simulink model "quanser_aero_dynamics4"  (R2021a)
settings: Solver=ode1  StartTime=0.0  StopTime=inf  FixedStep=0.002  RelTol=1e-3  EnableMultiTasking=on
PreLoadFcn:
  | quanser_aero_pd_design;
undefined symbols (not defined in the file): Kc, Kr
libraries: quanser_aero x1
settings Model: SimulationMode=external  ExtModeTrigDuration=15000  Creator=MLevis  LastModifiedBy=Mechatronics
settings SolverCC: AlgebraicLoopSolver=TrustRegion  PositivePriorityOrder=on
settings DataIOCC: LimitDataPoints=on  SaveFormat=Array  ReturnWorkspaceOutputs=off
settings DebuggingCC: SolverPrmCheckMsg=warning  SFUnexpectedBacktrackingDiag=warning  SFNoUnconditionalDefaultTransitionDiag=warning  SFExecutionAtInitializationDiag=none  SFMachineParentedDataDiag=warning  ArithmeticOperatorsInVariantConditions=warning
settings ModelReferenceCC: PropagateSignalLabelsOutOfModel=off
settings SFSimCC: SimUseLocalCustomCode=off  CustomCodeUndefinedFunction=UseInterfaceOnly
settings RTWCC: Description=QUARC Win64 Target Using Toolchain  SystemTargetFile=quarc_win64.tlc  TemplateMakefile=quarc_default_tmf  RTWUseLocalCustomCode=off  Toolchain=QUARC win64 | nmake (64-bit Windows)  BuildConfiguration=Faster Runs
settings CodeAppCC: StateflowObjectComments=on
settings STFCustomTargetCC: ConcurrentExecutionCompliant=on  SystemTargetFile=quarc_win64.tlc
settings GRTTargetCC: TargetLangStandard=C89/C90 (ANSI)  ParMdlRefBuildCompliant=off  CompOptLevelCompliant=off  CombineOutputUpdateFcns=off  MatFileLogging=off  CPPClassGenCompliant=off  GRTInterface=on  ExtMode=on  ExtModeMexFile=quarc_comm
settings ConfigComp: CovMetricSettings=dw  CovSaveCumulativeToWorkspaceVar=on  CovSaveSingleToWorkspaceVar=on  CovExternalEMLEnable=off  CovSFcnEnable=off

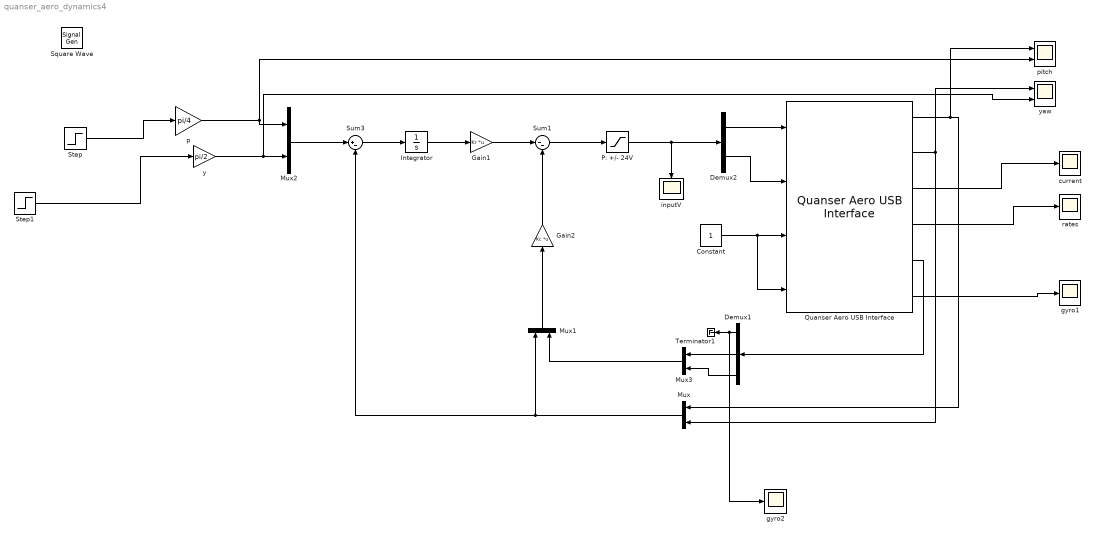
== system quanser_aero_dynamics4 ==
  Constant : Constant
  Demux1 : Demux  Outputs=3
  Demux2 : Demux  Outputs=2
  Gain1 : Gain  Gain=Kr  Multiplication=Matrix(K*u)
  Gain2 : Gain  Gain=Kc  Multiplication=Matrix(K*u)
  Integrator : Integrator
  Mux{,1..3} (4 alike) : Mux  Inputs=2
  P: +/- 24V : Saturate  UpperLimit=24  LowerLimit=-24
  Quanser Aero USB Interface : quanser_aero/Quanser Aero USB Interface  SystemSampleTime=-1  VariantActivationTime=update diagram  Latency=0  AutoFrameSizeCalculation=off
  "Square Wave " : SignalGenerator  WaveForm=square  Frequency=1/8
  Step : Step  Time=0  SampleTime=0
  Step1 : Step  Time=0  SampleTime=0
  Sum1 : Sum  Inputs=|--
  Sum3 : Sum  Inputs=|+-
  Terminator1 : Terminator
  current : Scope
  gyro1 : Scope
  gyro2 : Scope
  inputV : Scope
  p : Gain  Gain=pi/4
  pitch : Scope  NumInputPorts=2
  rates : Scope
  y : Gain  Gain=pi/2
  yaw : Scope  NumInputPorts=2
  wires:
  Mux2/1 -> Sum3/1
  Quanser Aero USB Interface/5 -> Demux1/1
  Quanser Aero USB Interface/4 -> rates/1
  Quanser Aero USB Interface/3 -> current/1
  Constant/1 -> Quanser Aero USB Interface/3, Quanser Aero USB Interface/4
  Quanser Aero USB Interface/6 -> gyro1/1
  Demux1/3 -> Mux3/2
  Demux1/2 -> Mux3/1
  Demux2/1 -> Quanser Aero USB Interface/1
  Demux2/2 -> Quanser Aero USB Interface/2
  P: +/- 24V/1 -> inputV/1, Demux2/1
  Quanser Aero USB Interface/1 -> pitch/1, Mux/1
  Quanser Aero USB Interface/2 -> yaw/1, Mux/2
  Mux/1 -> Sum3/2, Mux1/1
  p/1 -> Mux2/1, pitch/2
  y/1 -> yaw/2, Mux2/2
  Step/1 -> p/1
  Sum3/1 -> Integrator/1
  Integrator/1 -> Gain1/1
  Gain1/1 -> Sum1/1
  Sum1/1 -> P: +/- 24V/1
  Mux3/1 -> Mux1/2
  Mux1/1 -> Gain2/1
  Gain2/1 -> Sum1/2
  Demux1/1 -> gyro2/1, Terminator1/1
  Step1/1 -> y/1
